simulink model "Force_Control"  (R2020a)
settings: Solver=ode45  StartTime=0.0  StopTime=10  RelTol=1e-3
values from neighbouring files (symbols this model uses):
  B = 0.01    [Teleop_parameters.m]    (also in base.mat = 0.0517063081696; base_no_attrito.mat = 0; ci_siamo.mat = 0.0517063081696; force_control.mat = 0.0517063081696)
  Be = 10    [Teleop_parameters.m]    (also in base.mat = 0.5; base_no_attrito.mat = 0.5; ci_siamo.mat = 5; force_control.mat = 0.5)
  J = 0.010    (= 0.01)    [Teleop_parameters.m]    (also in base.mat = 0.0629265770424; base_no_attrito.mat = 0.0629265770424; ci_siamo.mat = 0.0629265770424; force_control.mat = 0.0629265770424)
  J_r = 0.1    [Teleop_parameters.m]    (also in base.mat = 0.0943898655636; base_no_attrito.mat = 0.0943898655636; ci_siamo.mat = 0.0629265770424; force_control.mat = 0.0943898655636)
  Ke = 2    [Teleop_parameters.m]    (also in base.mat = 10; base_no_attrito.mat = 10; ci_siamo.mat = 10; force_control.mat = 10)
  Kp_s = 200    [Teleop_parameters.m]    (also in base.mat = 1; base_no_attrito.mat = 1; ci_siamo.mat = 1; force_control.mat = 1)
  lArm_s = 0.1    [Teleop_parameters.m]    (also in base.mat; base_no_attrito.mat; ci_siamo.mat; force_control.mat)
  qe = 0.5    [Teleop_parameters.m]    (also in base.mat = 5; base_no_attrito.mat = 5; ci_siamo.mat; force_control.mat = 5)
settings Model: Creator=kriato  LastModifiedBy=giovanni

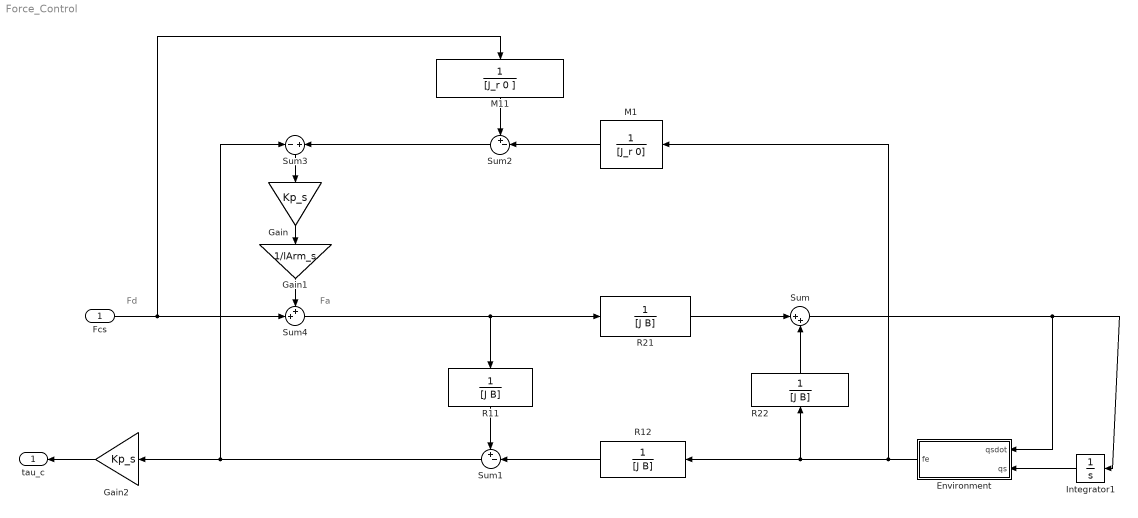
== system Force_Control ==
  note: Fa
  note: Fd
  Fcs : Inport
  Environment : Subsystem
  Gain : Gain  Gain=Kp_s
  Gain1 : Gain  Gain=1/lArm_s
  Gain2 : Gain  Gain=Kp_s
  Integrator1 : Integrator
  M1 : TransferFcn  Denominator=[J_r 0]
  M11 : TransferFcn  Denominator=[J_r 0 ]
  R{11..12,21..22} (4 alike) : TransferFcn  Denominator=[J B]
  Sum : Sum  Inputs=|++
  Sum1 : Sum  Inputs=+-|
  Sum2 : Sum  Inputs=+-|
  Sum3 : Sum  Inputs=-|+
  Sum4 : Sum  Inputs=++|
  tau_c : Outport
  wires:
  M1/1 -> Sum2/2
  Gain/1 -> Gain1/1
  Environment/1(fe) -> M1/1, R12/1, R22/1
  Sum/1 -> Integrator1/1, Environment/1(qsdot)
  Sum3/1 -> Gain/1
  Sum2/1 -> Sum3/2
  Sum4/1 -> R11/1, R21/1
  Gain1/1 -> Sum4/1
  R11/1 -> Sum1/1
  Gain2/1 -> tau_c/1
  R21/1 -> Sum/1
  M11/1 -> Sum2/1
  Fcs/1 -> M11/1, Sum4/2
  Sum1/1 -> Sum3/1, Gain2/1
  R12/1 -> Sum1/2
  R22/1 -> Sum/2
  Integrator1/1 -> Environment/2(qs)

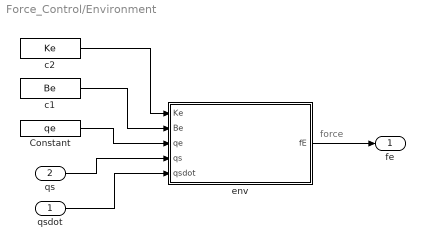
== system Force_Control/Environment ==
  note: force
  qsdot : Inport
  qs : Inport  Port=2
  Constant : Constant  Value=qe  SampleTime=0
  c1 : Constant  Value=Be  SampleTime=0
  c2 : Constant  Value=Ke  SampleTime=0
  env : MATLAB Function  TreatAsAtomicUnit=on
  fe : Outport  VectorParamsAs1DForOutWhenUnconnected=off
  wires:
  Constant/1 -> env/3(qe)
  c1/1 -> env/2(Be)
  c2/1 -> env/1(Ke)
  qs/1 -> env/4(qs)
  qsdot/1 -> env/5(qsdot)
  env/1(fE) -> fe/1

== matlab function Force_Control/Environment/env ==
  data: Ke input; Be input; qe input; qs input; fE output; qsdot input
function fE  = environment(Ke, Be, qe, qs, qsdot)
if qs > qe
   fE = Ke * (qs - qe) + Be * qsdot;
else
   fE = 0;
end
